simulink model "engine_model"  (R2023a)
settings: Solver=VariableStepAuto  StartTime=0.0  StopTime=10.0  RelTol=1e-3
settings Model: Creator=Pedro  LastModifiedBy=Pedro

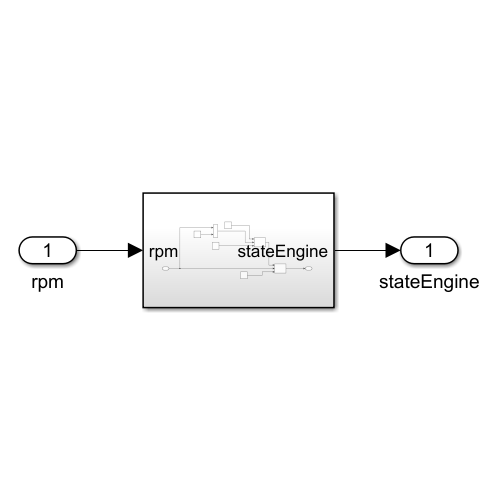
[thumbnail: Simulink's stored preview of the top-level diagram]
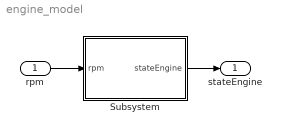
== system engine_model ==
  rpm : Inport
  Subsystem : Subsystem
  stateEngine : Outport
  wires:
  rpm/1 -> Subsystem/1(rpm)
  Subsystem/1(stateEngine) -> stateEngine/1

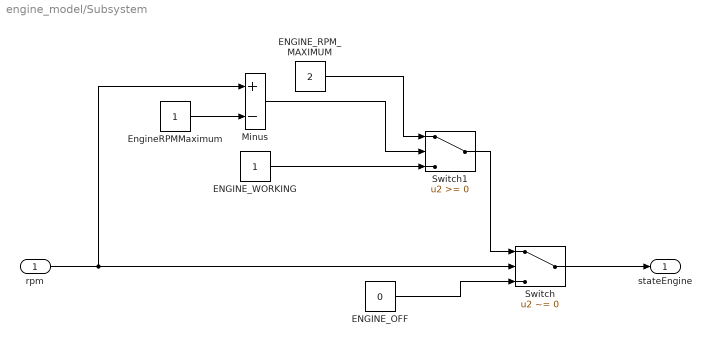
== system engine_model/Subsystem ==
  rpm : Inport
  ENGINE_OFF : Constant  Value=0
  ENGINE_RPM_MAXIMUM : Constant  Value=2
  ENGINE_WORKING : Constant
  EngineRPMMaximum : Constant
  Minus : Sum  Inputs=+-
  Switch : Switch  Criteria=u2 ~= 0  SaturateOnIntegerOverflow=off  InputSameDT=off
  Switch1 : Switch  SaturateOnIntegerOverflow=off  InputSameDT=off
  stateEngine : Outport
  wires:
  Switch1/1 -> Switch/1
  rpm/1 -> Switch/2, Minus/1
  ENGINE_RPM_MAXIMUM/1 -> Switch1/1
  ENGINE_WORKING/1 -> Switch1/3
  EngineRPMMaximum/1 -> Minus/2
  ENGINE_OFF/1 -> Switch/3
  Switch/1 -> stateEngine/1
  Minus/1 -> Switch1/2
